simulink model "PID_controller"  (R2020b)
settings: Solver=VariableStepAuto  StartTime=0.0  StopTime=10.0  RelTol=1e-3
model workspace (MAT data in the model file):
  Kd = Simulink.Parameter
  Kd.Value = 0.48976
  Kd.DataType = 'auto'
  Kd.Dimensions = [1 1]
  Ki = Simulink.Parameter
  Ki.Value = 97.11
  Ki.DataType = 'auto'
  Ki.Dimensions = [1 1]
  Kp = Simulink.Parameter
  Kp.Value = 4810.143
  Kp.DataType = 'auto'
  Kp.Dimensions = [1 1]
  N = Simulink.Parameter
  N.Value = 100000
  N.DataType = 'auto'
  N.Dimensions = [1 1]
settings Model: DataDictionary=problem_4_motor.sldd  Creator=Yeshwanth  LastModifiedBy=Yeshwanth
settings DataIOCC: SaveOutput=off  SaveTime=off

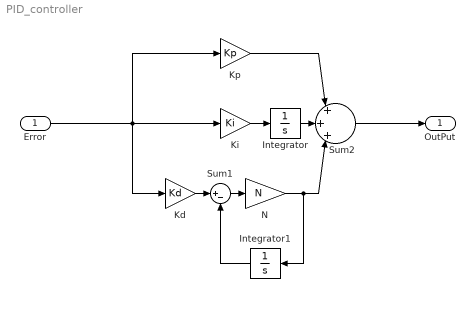
== system PID_controller ==
  Error : Inport  OutDataTypeStr=double  PortDimensions=1  SampleTime=0
  Integrator : Integrator
  Integrator1 : Integrator
  Kd : Gain  Gain=Kd
  Ki : Gain  Gain=Ki
  Kp : Gain  Gain=Kp
  N : Gain  Gain=N
  Sum1 : Sum  Inputs=|+-
  Sum2 : Sum  Inputs=|+|+|+|
  OutPut : Outport  OutDataTypeStr=double  PortDimensions=1  SampleTime=0
  wires:
  Kd/1 -> Sum1/1
  Error/1 -> Ki/1, Kp/1, Kd/1
  Ki/1 -> Integrator/1
  Kp/1 -> Sum2/1
  Integrator/1 -> Sum2/2
  Sum1/1 -> N/1
  Sum2/1 -> OutPut/1
  N/1 -> Integrator1/1, Sum2/3
  Integrator1/1 -> Sum1/2
